simulink model "receive"  (Simulink 7.8)
settings: Solver=ode45  StartTime=0.0  StopTime=100  RelTol=1e-3
libraries: simulink x1
settings Model: Creator=TGANJINE  LastModifiedBy=tganjine

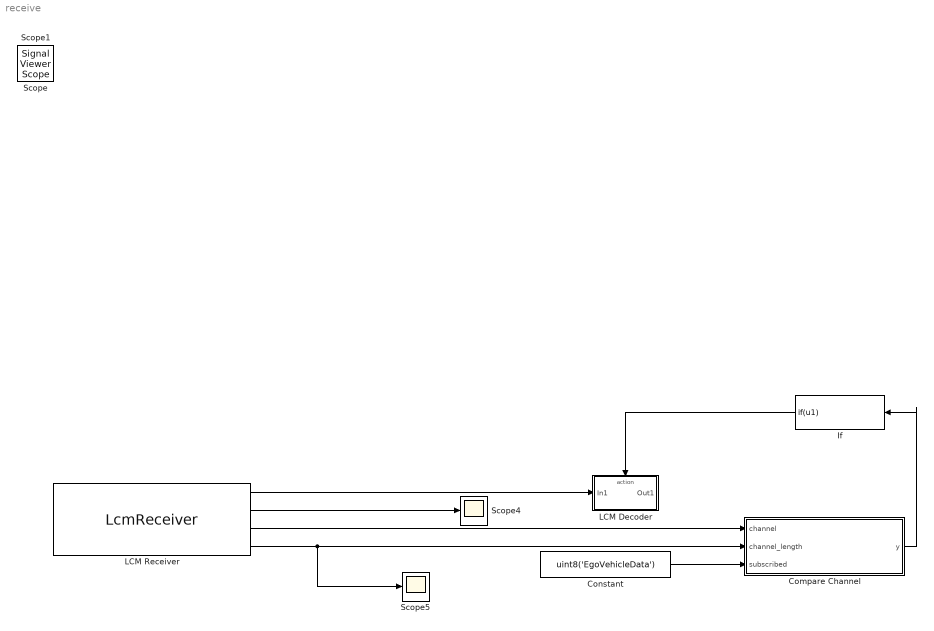
== system receive ==
  Compare Channel : MATLAB Function  TreatAsAtomicUnit=on
  Constant : Constant  Value=uint8('EgoVehicleData')
  If : If  IfExpression=u1  ShowElse=off
  LCM Decoder : Subsystem  TreatAsAtomicUnit=on
  LCM Receiver : S-Function  FunctionName=LcmReceiver  Parameters=Address, Port, Channel, MaxMessageSize  EnableBusSupport=off  mask(LcmReceiver){Address=127.0.0.1, Port=7700, Channel=.*, MaxMessageSize=10240}
      mask prompts: Channel "Channel name"; MaxMessageSize "Maximal message size"
      mask help:
      | This block acts as receiver for LCM messages over TCP. It also doubles as log time sychronizer together with Autonomos framework/Log Timer.
      | The messages for the log time synchronization are send inband with an LCM type.
      |
      | If it cannot connect to the server it will error out. If it can connect, but does not receive any data, it will block.
      | If it blocks, you can stop the TCPService to stop the blocking receive.
      mask Display:
      | fprintf('Receiver/LogTimer\n%s:%s\n%s', Address, Port, Channel)
      | port_label('output', 1, 'data')
      | port_label('output', 2, 'data_length')
      | port_label('output', 3, 'channel')
      | port_label('output', 4, 'channel_length')
  Scope4 : Scope
      settings: YMin=0  YMax=7500  SaveName=ScopeData3
  Scope5 : Scope
      settings: SaveName=ScopeData4
  Scope : SignalViewerScope  IOType=viewer  RefreshTime=0.035000
  Scope1 : SignalViewerScope  IOType=viewer  RefreshTime=0.035000
  wires:
  LCM Receiver/2 -> Scope4/1
  LCM Receiver/4 -> Scope5/1, Compare Channel/2(channel_length)
  LCM Receiver/1 -> LCM Decoder/1(In1)
  LCM Receiver/3 -> Compare Channel/1(channel)
  Constant/1 -> Compare Channel/3(subscribed)
  Compare Channel/1(y) -> If/1
  If/1 -> LCM Decoder/Action

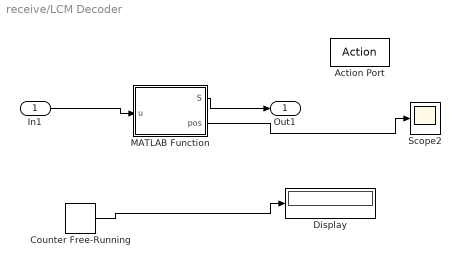
== system receive/LCM Decoder ==
  In1 : Inport
  Action Port : ActionPort  ActionType=then
  Counter Free-Running : simulink/Sources/Counter Free-Running  NumBits=16  tsamp=-1
  Display : Display
  MATLAB Function : MATLAB Function  TreatAsAtomicUnit=on
  Scope2 : Scope
      settings: YMax=80
  Out1 : Outport
  wires:
  In1/1 -> MATLAB Function/1(u)
  MATLAB Function/1(S) -> Out1/1
  Counter Free-Running/1 -> Display/1
  MATLAB Function/2(pos) -> Scope2/1

== matlab function Compare Channel ==
  data: channel input double; y output double; channel_length input double; subscribed input double
function y = fcn(channel, channel_length, subscribed)
%#codegen
y = isequal(channel(1:channel_length), subscribed(:));

== matlab function LCM Decoder/MATLAB Function ==
  data: u input double; S output Bus: busObjEgoVehicleData; pos output double
function [S, pos] = fcn(u)
%#codegen
y = busObjEgoVehicleData_new();
[pos, S] = busObjEgoVehicleData_decode(u, 1, length(u), y);
